simulink model "untitled_model"  (R2021a)
settings: Solver=VariableStepAuto  StartTime=0.0  StopTime=50  RelTol=1e-3
undefined symbols (not defined in the file): a, b
settings Model: Creator=mavolery  LastModifiedBy=padlewsk
settings SolverCC: AlgebraicLoopSolver=TrustRegion
settings DebuggingCC: SFMachineParentedDataDiag=warning

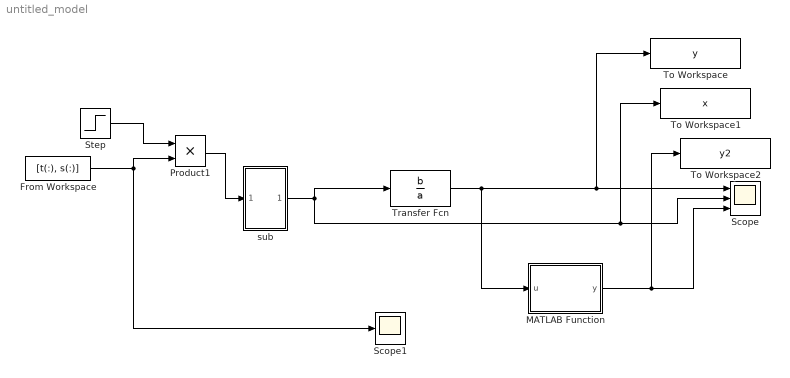
== system untitled_model ==
  From Workspace : FromWorkspace  VariableName=[t(:), s(:)]  SampleTime=0.01  OutputAfterFinalValue=Holding final value
  MATLAB Function : MATLAB Function  TreatAsAtomicUnit=on
  Product1 : Product
  Scope : Scope  NumInputPorts=3
  Scope1 : Scope
  Step : Step  SampleTime=0
  To Workspace : ToWorkspace  VariableName=y  SampleTime=-1
      settings: Save2DSignal=2-D array (concatenate along first dimension)
  To Workspace1 : ToWorkspace  VariableName=x  SampleTime=-1
      settings: Save2DSignal=2-D array (concatenate along first dimension)
  To Workspace2 : ToWorkspace  VariableName=y2  SampleTime=-1
      settings: Save2DSignal=2-D array (concatenate along first dimension)
  Transfer Fcn : TransferFcn  Numerator=b  Denominator=a
  sub : Subsystem
  wires:
  Transfer Fcn/1 -> MATLAB Function/1(u), To Workspace/1, Scope/1
  MATLAB Function/1(y) -> To Workspace2/1, Scope/3
  Step/1 -> Product1/1
  From Workspace/1 -> Product1/2, Scope1/1
  sub/1(Out1) -> Transfer Fcn/1, To Workspace1/1, Scope/2
  Product1/1 -> sub/1(In1)

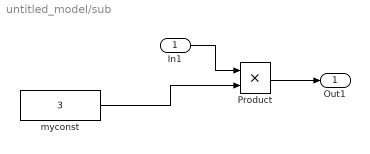
== system untitled_model/sub ==
  In1 : Inport
  Product : Product
  myconst : Constant  Value=3
  Out1 : Outport
  wires:
  myconst/1 -> Product/2
  Product/1 -> Out1/1
  In1/1 -> Product/1

== matlab function untitled_model/MATLAB Function ==
  data: u input; y output
function y = fcn(u)
y = u^2;
